simulink model "matlab1"  (R2019a)
settings: Solver=FixedStepAuto  StartTime=0.0  StopTime=inf  RelTol=1e-3  EnableMultiTasking=on
libraries: vexarmcortexlib x25
settings Model: Creator=maxim  LastModifiedBy=Allen
settings DataIOCC: LimitDataPoints=on  SignalLoggingSaveFormat=ModelDataLogs  ReturnWorkspaceOutputs=off
settings OptimizationCC: ExpressionDepthLimit=2147483647  LifeSpan=Inf  MaxStackSize=64
settings DebuggingCC: UnderspecifiedInitializationDetection=Classic  MergeDetectMultiDrivingBlocksExec=none  InheritedTsInSrcMsg=none  FcnCallInpInsideContextMsg=warning  UnconnectedInputMsg=none  UnconnectedOutputMsg=none  StateNameClashWarn=warning  SFUnexpectedBacktrackingDiag=warning  SFNoUnconditionalDefaultTransitionDiag=warning  SFExecutionAtInitializationDiag=none  ArithmeticOperatorsInVariantConditions=warning
settings HardwareCC: ProdBitPerPointer=32  ProdBitPerSizeT=32  ProdBitPerPtrDiffT=32  ProdLargestAtomicInteger=Long  ProdLargestAtomicFloat=Double  ProdIntDivRoundTo=Undefined  ProdWordSize=32  ProdHWDeviceType=ARM Compatible->ARM Cortex  UseEmbeddedCoderFeatures=off
settings ModelReferenceCC: PropagateSignalLabelsOutOfModel=off
settings SFSimCC: MATLABDynamicMemAlloc=off
settings RTWCC: SystemTargetFile=ert.tlc  HardwareBoard=ARM Cortex-based VEX Microcontroller  TemplateMakefile=ert_default_tmf  Toolchain=GNU Tools for VEX ARM Cortex
settings CodeAppCC: IgnoreCustomStorageClasses=off  CustomSymbolStrType=$N$R$M  StateflowObjectComments=on  InternalIdentifier=Classic
settings ERTTargetCC: CodeReplacementLibrary=GCC ARM Cortex-M3  MultiwordLength=2048  SupportNonInlinedSFcns=on  ConvertIfToSwitch=off  SuppressUnreachableDefaultCases=off

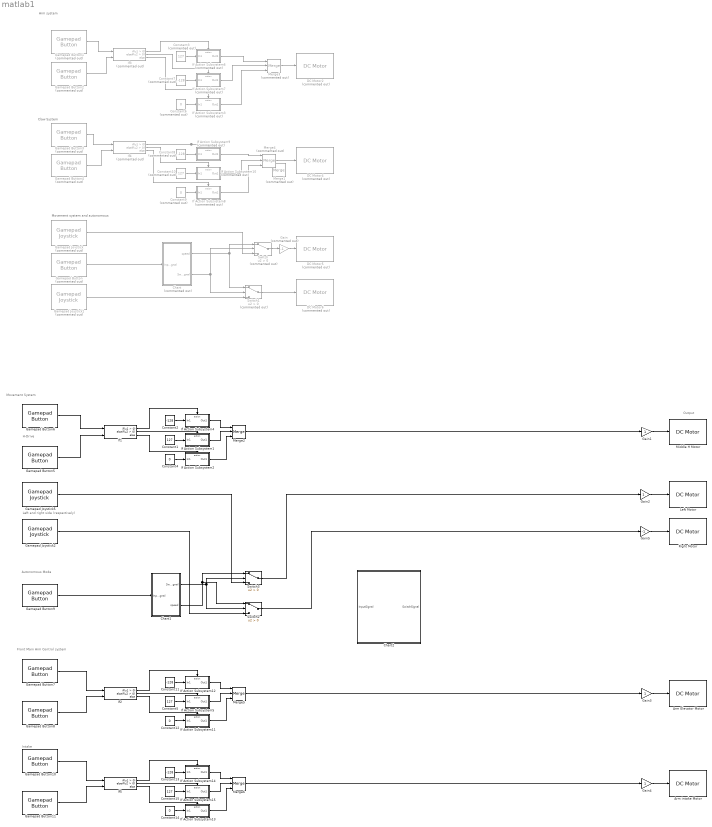
== system matlab1 ==
  note: Output
  note: Intake
  note: Left and right side (respectively)
  note: H-Drive
  note: Autonomous Mode
  note: Front Main Arm Control system
  note: Movement System
  note: Arm system
  note: Claw System
  note: Movement system and autonomous
  Arm Elevator Motor : vexarmcortexlib/Actuators/DC Motor  motor=5  scaleFactor=1/13.5  SimulationOut=off
      settings: SourceProductName=Simulink Coder Support Package for ARM Cortex-based VEX Microcontroller  SourceProductBaseCode=EC_VEX_MICRO
  Arm intake Motor : vexarmcortexlib/Actuators/DC Motor  motor=5  scaleFactor=1/13.5  SimulationOut=off
      settings: SourceProductName=Simulink Coder Support Package for ARM Cortex-based VEX Microcontroller  SourceProductBaseCode=EC_VEX_MICRO
  Chart : Stateflow chart  Commented=on  BlockKeywords=__PRM__SERIALIZED__DATA__:Stateflow Chart,Stateflow Diagram  TreatAsAtomicUnit=on
  Chart1 : Stateflow chart  BlockKeywords=__PRM__SERIALIZED__DATA__:Stateflow Chart,Stateflow Diagram  TreatAsAtomicUnit=on
  Chart2 : Stateflow chart  BlockKeywords=__PRM__SERIALIZED__DATA__:Stateflow Chart,Stateflow Diagram  TreatAsAtomicUnit=on
  Constant1 : Constant  Value=127
  Constant10 : Constant  Commented=on  Value=127
  Constant11 : Constant  Value=-128
  Constant12 : Constant  Value=0
  Constant13 : Constant  Value=-128
  Constant14 : Constant  Value=0
  Constant15 : Constant  Value=127
  Constant2 : Constant  Value=-128
  Constant3 : Constant  Commented=on  Value=127
  Constant4 : Constant  Value=0
  Constant5 : Constant  Value=127
  Constant6 : Constant  Commented=on  Value=0
  Constant7 : Constant  Commented=on  Value=-128
  Constant8 : Constant  Commented=on  Value=-128
  Constant9 : Constant  Commented=on  Value=0
  DC Motor2 : vexarmcortexlib/Actuators/DC Motor  Commented=on  motor=5  scaleFactor=1/13.5  SimulationOut=off
      settings: SourceProductName=Simulink Coder Support Package for ARM Cortex-based VEX Microcontroller  SourceProductBaseCode=EC_VEX_MICRO
  DC Motor4 : vexarmcortexlib/Actuators/DC Motor  Commented=on  motor=6  scaleFactor=1/13.5  SimulationOut=off
      settings: SourceProductName=Simulink Coder Support Package for ARM Cortex-based VEX Microcontroller  SourceProductBaseCode=EC_VEX_MICRO
  DC Motor5 : vexarmcortexlib/Actuators/DC Motor  Commented=on  motor=1  scaleFactor=1/13.5  SimulationOut=off
      settings: SourceProductName=Simulink Coder Support Package for ARM Cortex-based VEX Microcontroller  SourceProductBaseCode=EC_VEX_MICRO
  DC Motor6 : vexarmcortexlib/Actuators/DC Motor  Commented=on  motor=10  scaleFactor=1/13.5  SimulationOut=off
      settings: SourceProductName=Simulink Coder Support Package for ARM Cortex-based VEX Microcontroller  SourceProductBaseCode=EC_VEX_MICRO
  Gain : Gain  Commented=on  Gain=-1
  Gain{1..4} (4 alike) : Gain
  Gain5 : Gain  Gain=-1
  Gamepad Button : vexarmcortexlib/Gamepad/Gamepad Button  Commented=on  joystick=1  chan=7  button56=Down  button78=Down  SimulationIn=off  SampleTime=0.02
      settings: SourceProductName=Simulink Coder Support Package for ARM Cortex-based VEX Microcontroller  SourceProductBaseCode=EC_VEX_MICRO
  Gamepad Button1 : vexarmcortexlib/Gamepad/Gamepad Button  Commented=on  joystick=1  chan=5  button56=Up  button78=Down  SimulationIn=off  SampleTime=0.02
      settings: SourceProductName=Simulink Coder Support Package for ARM Cortex-based VEX Microcontroller  SourceProductBaseCode=EC_VEX_MICRO
  Gamepad Button10 : vexarmcortexlib/Gamepad/Gamepad Button  joystick=1  chan=7  button56=Up  button78=Up  SimulationIn=off  SampleTime=0.02
      settings: SourceProductName=Simulink Coder Support Package for ARM Cortex-based VEX Microcontroller  SourceProductBaseCode=EC_VEX_MICRO
  Gamepad Button11 : vexarmcortexlib/Gamepad/Gamepad Button  joystick=1  chan=7  button56=Up  button78=Left  SimulationIn=off  SampleTime=0.02
      settings: SourceProductName=Simulink Coder Support Package for ARM Cortex-based VEX Microcontroller  SourceProductBaseCode=EC_VEX_MICRO
  Gamepad Button2 : vexarmcortexlib/Gamepad/Gamepad Button  Commented=on  joystick=1  chan=5  button56=Down  button78=Down  SimulationIn=off  SampleTime=0.02
      settings: SourceProductName=Simulink Coder Support Package for ARM Cortex-based VEX Microcontroller  SourceProductBaseCode=EC_VEX_MICRO
  Gamepad Button3 : vexarmcortexlib/Gamepad/Gamepad Button  Commented=on  joystick=1  chan=6  button56=Up  button78=Up  SimulationIn=off  SampleTime=0.02
      settings: SourceProductName=Simulink Coder Support Package for ARM Cortex-based VEX Microcontroller  SourceProductBaseCode=EC_VEX_MICRO
  Gamepad Button4 : vexarmcortexlib/Gamepad/Gamepad Button  Commented=on  joystick=1  chan=6  button56=Down  button78=Down  SimulationIn=off  SampleTime=0.02
      settings: SourceProductName=Simulink Coder Support Package for ARM Cortex-based VEX Microcontroller  SourceProductBaseCode=EC_VEX_MICRO
  Gamepad Button5 : vexarmcortexlib/Gamepad/Gamepad Button  joystick=1  chan=6  button56=Up  button78=Down  SimulationIn=off  SampleTime=0.02
      settings: SourceProductName=Simulink Coder Support Package for ARM Cortex-based VEX Microcontroller  SourceProductBaseCode=EC_VEX_MICRO
  Gamepad Button6 : vexarmcortexlib/Gamepad/Gamepad Button  joystick=1  chan=5  button56=Up  button78=Down  SimulationIn=off  SampleTime=0.02
      settings: SourceProductName=Simulink Coder Support Package for ARM Cortex-based VEX Microcontroller  SourceProductBaseCode=EC_VEX_MICRO
  Gamepad Button7 : vexarmcortexlib/Gamepad/Gamepad Button  joystick=1  chan=8  button56=Up  button78=Up  SimulationIn=off  SampleTime=0.02
      settings: SourceProductName=Simulink Coder Support Package for ARM Cortex-based VEX Microcontroller  SourceProductBaseCode=EC_VEX_MICRO
  Gamepad Button8 : vexarmcortexlib/Gamepad/Gamepad Button  joystick=1  chan=8  button56=Up  button78=Left  SimulationIn=off  SampleTime=0.02
      settings: SourceProductName=Simulink Coder Support Package for ARM Cortex-based VEX Microcontroller  SourceProductBaseCode=EC_VEX_MICRO
  Gamepad Button9 : vexarmcortexlib/Gamepad/Gamepad Button  joystick=1  chan=7  button56=Down  button78=Down  SimulationIn=off  SampleTime=0.02
      settings: SourceProductName=Simulink Coder Support Package for ARM Cortex-based VEX Microcontroller  SourceProductBaseCode=EC_VEX_MICRO
  Gamepad Joystick : vexarmcortexlib/Gamepad/Gamepad Joystick  Commented=on  joystick=1  chan=2  SimulationIn=off  SampleTime=0.02
      settings: SourceProductName=Simulink Coder Support Package for ARM Cortex-based VEX Microcontroller  SourceProductBaseCode=EC_VEX_MICRO
  Gamepad Joystick1 : vexarmcortexlib/Gamepad/Gamepad Joystick  Commented=on  joystick=1  chan=3  SimulationIn=off  SampleTime=0.02
      settings: SourceProductName=Simulink Coder Support Package for ARM Cortex-based VEX Microcontroller  SourceProductBaseCode=EC_VEX_MICRO
  Gamepad Joystick2 : vexarmcortexlib/Gamepad/Gamepad Joystick  joystick=1  chan=2  SimulationIn=off  SampleTime=0.02
      settings: SourceProductName=Simulink Coder Support Package for ARM Cortex-based VEX Microcontroller  SourceProductBaseCode=EC_VEX_MICRO
  Gamepad Joystick5 : vexarmcortexlib/Gamepad/Gamepad Joystick  joystick=1  chan=3  SimulationIn=off  SampleTime=0.02
      settings: SourceProductName=Simulink Coder Support Package for ARM Cortex-based VEX Microcontroller  SourceProductBaseCode=EC_VEX_MICRO
  If Action Subsystem1 : Subsystem  TreatAsAtomicUnit=on
  If Action Subsystem10 : Subsystem  Commented=on  TreatAsAtomicUnit=on
  If Action Subsystem11 : Subsystem  TreatAsAtomicUnit=on
  If Action Subsystem12 : Subsystem  TreatAsAtomicUnit=on
  If Action Subsystem13 : Subsystem  TreatAsAtomicUnit=on
  If Action Subsystem14 : Subsystem  TreatAsAtomicUnit=on
  If Action Subsystem15 : Subsystem  TreatAsAtomicUnit=on
  If Action Subsystem2 : Subsystem  TreatAsAtomicUnit=on
  If Action Subsystem3 : Subsystem  Commented=on  TreatAsAtomicUnit=on
  If Action Subsystem4 : Subsystem  TreatAsAtomicUnit=on
  If Action Subsystem5 : Subsystem  TreatAsAtomicUnit=on
  If Action Subsystem6 : Subsystem  Commented=on  TreatAsAtomicUnit=on
  If Action Subsystem7 : Subsystem  Commented=on  TreatAsAtomicUnit=on
  If Action Subsystem8 : Subsystem  Commented=on  TreatAsAtomicUnit=on
  If Action Subsystem9 : Subsystem  Commented=on  TreatAsAtomicUnit=on
  If1 : If  NumInputs=2  ElseIfExpressions=u2 > 0
  If2 : If  NumInputs=2  ElseIfExpressions=u2 > 0
  If3 : If  Commented=on  NumInputs=2  ElseIfExpressions=u2 > 0
  If4 : If  Commented=on  NumInputs=2  ElseIfExpressions=u2 > 0
  If5 : If  NumInputs=2  ElseIfExpressions=u2 > 0
  "Left Motor " : vexarmcortexlib/Actuators/DC Motor  motor=4  scaleFactor=1/13.5  SimulationOut=off
      settings: SourceProductName=Simulink Coder Support Package for ARM Cortex-based VEX Microcontroller  SourceProductBaseCode=EC_VEX_MICRO
  Merge1 : Merge  Commented=on  Inputs=3
  Merge2 : Merge  Inputs=3
  Merge3 : Merge  Commented=on  Inputs=3
  Merge4 : Merge  Commented=on  Inputs=3
  Merge5 : Merge  Inputs=3
  Merge6 : Merge  Inputs=3
  Middle H Motor : vexarmcortexlib/Actuators/DC Motor  motor=3  scaleFactor=1/13.5  SimulationOut=off
      settings: SourceProductName=Simulink Coder Support Package for ARM Cortex-based VEX Microcontroller  SourceProductBaseCode=EC_VEX_MICRO
  Right Motor : vexarmcortexlib/Actuators/DC Motor  motor=2  scaleFactor=1/13.5  SimulationOut=off
      settings: SourceProductName=Simulink Coder Support Package for ARM Cortex-based VEX Microcontroller  SourceProductBaseCode=EC_VEX_MICRO
  Switch : Switch  Commented=on  Criteria=u2 > Threshold
  Switch1 : Switch  Commented=on  Criteria=u2 > Threshold
  Switch2 : Switch  Criteria=u2 > Threshold
  Switch3 : Switch  Criteria=u2 > Threshold
  wires:
  Gamepad Joystick/1 -> Switch/3
  Gain/1 -> DC Motor5/1
  Gamepad Joystick1/1 -> Switch1/3
  Gamepad Button1/1 -> If3/1
  Gamepad Button2/1 -> If3/2
  If Action Subsystem6/1(Out1) -> Merge3/1
  If Action Subsystem3/1(Out1) -> Merge3/3
  Constant3/1 -> If Action Subsystem6/1(In1)
  If3/3 -> If Action Subsystem3/Action
  Constant6/1 -> If Action Subsystem3/1(In1)
  If3/1 -> If Action Subsystem6/Action
  Constant7/1 -> If Action Subsystem7/1(In1)
  If3/2 -> If Action Subsystem7/Action
  If Action Subsystem7/1(Out1) -> Merge3/2
  Merge3/1 -> DC Motor2/1
  Constant10/1 -> If Action Subsystem10/1(In1)
  If Action Subsystem10/1(Out1) -> Merge4/2
  If4/1 -> If Action Subsystem9/Action
  Constant8/1 -> If Action Subsystem9/1(In1)
  If4/3 -> If Action Subsystem8/Action
  If Action Subsystem8/1(Out1) -> Merge4/3
  Constant9/1 -> If Action Subsystem8/1(In1)
  If4/2 -> If Action Subsystem10/Action
  Merge4/1 -> DC Motor4/1
  Gamepad Button4/1 -> If4/2
  Gamepad Button3/1 -> If4/1
  If Action Subsystem9/1(Out1) -> Merge4/1
  Chart/1(speed) -> Switch1/1, Switch/1
  Chart/2(SwitchSignal) -> Switch/2, Switch1/2
  Switch1/1 -> DC Motor6/1
  Switch/1 -> Gain/1
  Gamepad Button/1 -> Chart/1(InputSignal)
  Gain1/1 -> Middle H Motor/1
  Gain5/1 -> Right Motor/1
  Gain2/1 -> "Left Motor "/1
  Gamepad Joystick2/1 -> Switch2/3
  Gamepad Joystick5/1 -> Switch3/3
  Merge2/1 -> Gain1/1
  Gamepad Button6/1 -> If1/1
  Gamepad Button5/1 -> If1/2
  Constant2/1 -> If Action Subsystem4/1(In1)
  If1/3 -> If Action Subsystem2/Action
  Constant1/1 -> If Action Subsystem1/1(In1)
  Constant4/1 -> If Action Subsystem2/1(In1)
  If1/2 -> If Action Subsystem1/Action
  If1/1 -> If Action Subsystem4/Action
  If Action Subsystem4/1(Out1) -> Merge2/1
  If Action Subsystem1/1(Out1) -> Merge2/2
  If Action Subsystem2/1(Out1) -> Merge2/3
  Gamepad Button9/1 -> Chart1/1(InputSignal)
  Chart1/2(speed) -> Switch2/1, Switch3/1
  Chart1/1(SwitchSignal) -> Switch2/2, Switch3/2
  Switch2/1 -> Gain5/1
  Switch3/1 -> Gain2/1
  Merge5/1 -> Gain3/1
  Constant12/1 -> If Action Subsystem11/1(In1)
  If2/1 -> If Action Subsystem12/Action
  Constant11/1 -> If Action Subsystem12/1(In1)
  If Action Subsystem11/1(Out1) -> Merge5/3
  If2/3 -> If Action Subsystem11/Action
  If Action Subsystem12/1(Out1) -> Merge5/1
  Constant5/1 -> If Action Subsystem5/1(In1)
  If2/2 -> If Action Subsystem5/Action
  Gain3/1 -> Arm Elevator Motor/1
  If Action Subsystem5/1(Out1) -> Merge5/2
  Gamepad Button7/1 -> If2/1
  Gamepad Button8/1 -> If2/2
  If5/1 -> If Action Subsystem14/Action
  Gamepad Button11/1 -> If5/2
  Gain4/1 -> Arm intake Motor/1
  If Action Subsystem15/1(Out1) -> Merge6/2
  Constant15/1 -> If Action Subsystem15/1(In1)
  If Action Subsystem14/1(Out1) -> Merge6/1
  If5/3 -> If Action Subsystem13/Action
  Gamepad Button10/1 -> If5/1
  Merge6/1 -> Gain4/1
  Constant13/1 -> If Action Subsystem14/1(In1)
  If Action Subsystem13/1(Out1) -> Merge6/3
  Constant14/1 -> If Action Subsystem13/1(In1)
  If5/2 -> If Action Subsystem15/Action

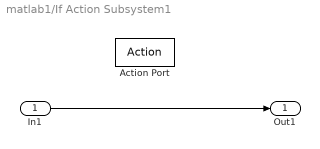
== system matlab1/If Action Subsystem1 ==
  In1 : Inport
  Action Port : ActionPort  ActionPortLabel=elseif(u2 > 0)
  Out1 : Outport  InitialOutput=127
  wires:
  In1/1 -> Out1/1

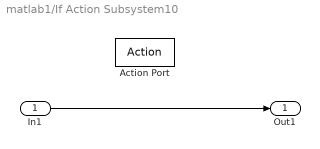
== system matlab1/If Action Subsystem10 ==
  In1 : Inport
  Action Port : ActionPort  ActionPortLabel=elseif(u2 > 0)
  Out1 : Outport  InitialOutput=127
  wires:
  In1/1 -> Out1/1

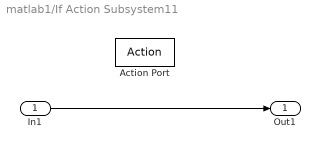
== system matlab1/If Action Subsystem11 ==
  In1 : Inport
  Action Port : ActionPort  ActionPortLabel=else
  Out1 : Outport
  wires:
  In1/1 -> Out1/1

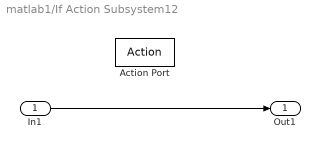
== system matlab1/If Action Subsystem12 ==
  In1 : Inport
  Action Port : ActionPort  ActionPortLabel=if(u1 > 0)
  Out1 : Outport  InitialOutput=127
  wires:
  In1/1 -> Out1/1

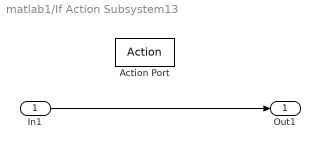
== system matlab1/If Action Subsystem13 ==
  In1 : Inport
  Action Port : ActionPort  ActionPortLabel=else
  Out1 : Outport
  wires:
  In1/1 -> Out1/1

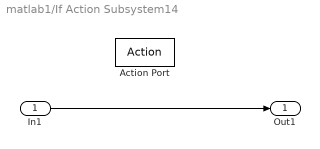
== system matlab1/If Action Subsystem14 ==
  In1 : Inport
  Action Port : ActionPort  ActionPortLabel=if(u1 > 0)
  Out1 : Outport  InitialOutput=127
  wires:
  In1/1 -> Out1/1

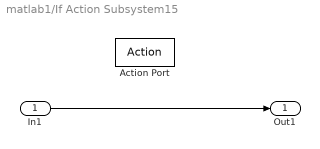
== system matlab1/If Action Subsystem15 ==
  In1 : Inport
  Action Port : ActionPort  ActionPortLabel=elseif(u2 > 0)
  Out1 : Outport  InitialOutput=127
  wires:
  In1/1 -> Out1/1

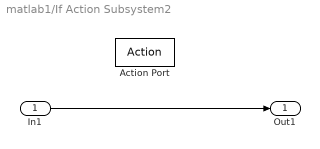
== system matlab1/If Action Subsystem2 ==
  In1 : Inport
  Action Port : ActionPort  ActionPortLabel=else
  Out1 : Outport
  wires:
  In1/1 -> Out1/1

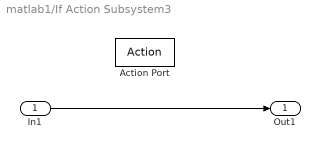
== system matlab1/If Action Subsystem3 ==
  In1 : Inport
  Action Port : ActionPort  ActionPortLabel=else
  Out1 : Outport
  wires:
  In1/1 -> Out1/1

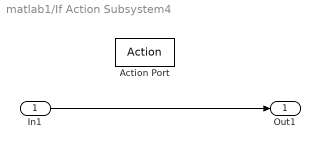
== system matlab1/If Action Subsystem4 ==
  In1 : Inport
  Action Port : ActionPort  ActionPortLabel=if(u1 > 0)
  Out1 : Outport  InitialOutput=127
  wires:
  In1/1 -> Out1/1

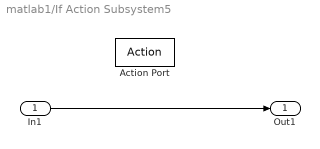
== system matlab1/If Action Subsystem5 ==
  In1 : Inport
  Action Port : ActionPort  ActionPortLabel=elseif(u2 > 0)
  Out1 : Outport  InitialOutput=127
  wires:
  In1/1 -> Out1/1

== system matlab1/If Action Subsystem6 ==
  In1 : Inport
  Action Port : ActionPort  ActionPortLabel=if(u1 > 0)
  Out1 : Outport  InitialOutput=127
  wires:
  In1/1 -> Out1/1

== system matlab1/If Action Subsystem7 ==
  In1 : Inport
  Action Port : ActionPort  ActionPortLabel=elseif(u2 > 0)
  Out1 : Outport  InitialOutput=127
  wires:
  In1/1 -> Out1/1

== system matlab1/If Action Subsystem8 ==
  In1 : Inport
  Action Port : ActionPort  ActionPortLabel=else
  Out1 : Outport
  wires:
  In1/1 -> Out1/1

== system matlab1/If Action Subsystem9 ==
  In1 : Inport
  Action Port : ActionPort  ActionPortLabel=if(u1 > 0)
  Out1 : Outport  InitialOutput=127
  wires:
  In1/1 -> Out1/1

== stateflow chart matlab1/Chart1 ==
  state Start
    during:
    SwitchSignal = 0;
  state Push_Backwards
    during:
    speed=-128;
  state Halt
    during:
    speed=0;
  state Push_Forward
    during:
    speed=127;
    SwitchSignal = 1;
  state Stop
    during:
    speed=0;
    SwitchSignal = 0;
  (default) -> Start : {speed = 0}
  Stop -> Start : after(0.1,sec)
  Start -> Push_Forward : [InputSignal >0]
  Halt -> Push_Backwards : after(3,sec)
  Push_Forward -> Halt : after(2,sec)
  Push_Backwards -> Stop : after(5,sec)
  data: SwitchSignal output; InputSignal input; speed output

== stateflow chart matlab1/Chart2 ==
  state CollectSoccerBalls
    during:
  state DepositSoccerBalls
    during:
  state DepositSoccerAndFootballs
    during:
  state CollectBaseballsAndFootballs
    during:
  state CollectBasketballs
    during:
  state DepositBasketballs
    during:
  state End
    during:
  CollectSoccerBalls -> DepositSoccerBalls
  (default) -> CollectSoccerBalls : [InputSignal >0]
  DepositSoccerBalls -> CollectBaseballsAndFootballs
  CollectBaseballsAndFootballs -> DepositSoccerAndFootballs
  DepositSoccerAndFootballs -> CollectBasketballs
  CollectBasketballs -> DepositBasketballs
  DepositBasketballs -> End
  data: SwitchSignal output; InputSignal input

== stateflow chart matlab1/Chart ==
  state Start
    during:
    SwitchSignal = 0;
  state Push_Backwards
    during:
    speed=-128;
  state Halt
    during:
    speed=0;
  state Push_Forward
    during:
    speed=127;
    SwitchSignal = 1;
  state Stop
    during:
    speed=0;
    SwitchSignal = 0;
  (default) -> Start : {speed = 0}
  Stop -> Start : after(0.1,sec)
  Start -> Push_Forward : [InputSignal >0]
  Halt -> Push_Backwards : after(3,sec)
  Push_Forward -> Halt : after(2,sec)
  Push_Backwards -> Stop : after(5,sec)
  data: speed output; SwitchSignal output; InputSignal input
